simulink model "Non_linear_model_step_response_small_large"  (R2021b)
settings: Solver=FixedStepAuto  StartTime=0.0  StopTime=30  FixedStep=0.001  RelTol=1e-3  EnableMultiTasking=on
undefined symbols (not defined in the file): F_js, F_s, LF, LF_j, LT_i, LT_ji, SF, SF_j, ST_i, ST_ji, T_is, T_jis, T_js, T_s
settings Model: Creator=Administrator  LastModifiedBy=Administrator

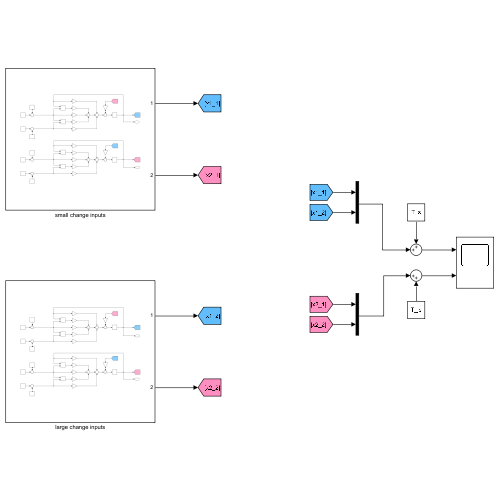
[thumbnail: Simulink's stored preview of the top-level diagram]
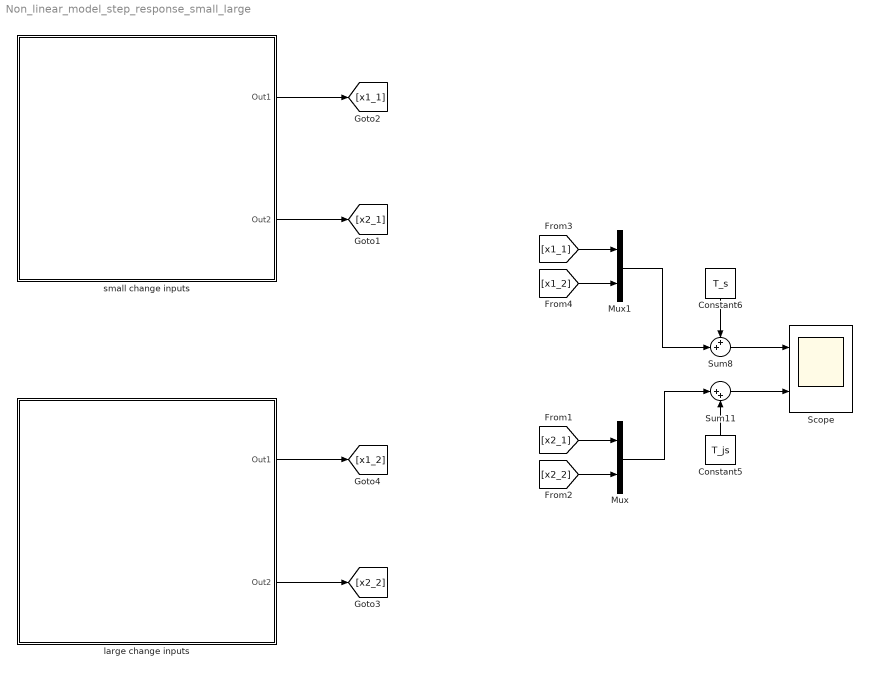
== system Non_linear_model_step_response_small_large ==
  Constant5 : Constant  Value=T_js
  Constant6 : Constant  Value=T_s
  Mux : Mux  Inputs=2
  Mux1 : Mux  Inputs=2
  Scope : Scope  NumInputPorts=2
  Sum11 : Sum  Inputs=|++
  Sum8 : Sum  Inputs=++|
  large change inputs : Subsystem
  small change inputs : Subsystem
  wires:
  Mux1/1 -> Sum8/2
  Sum8/1 -> Scope/1
  Sum11/1 -> Scope/2
  Mux/1 -> Sum11/1
  Constant5/1 -> Sum11/2
  Constant6/1 -> Sum8/1
  small change inputs/1(Out1) -> [x1_1]
  small change inputs/2(Out2) -> [x2_1]
  large change inputs/2(Out2) -> [x2_2]
  large change inputs/1(Out1) -> [x1_2]
  [x2_2] -> Mux/2
  [x2_1] -> Mux/1
  [x1_1] -> Mux1/1
  [x1_2] -> Mux1/2

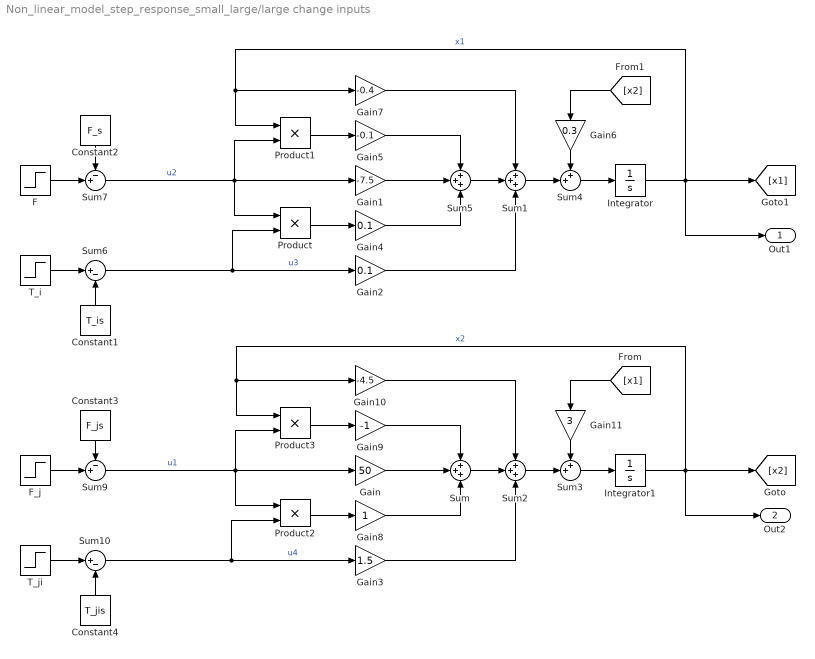
== system Non_linear_model_step_response_small_large/large change inputs ==
  Constant1 : Constant  Value=T_is
  Constant2 : Constant  Value=F_s
  Constant3 : Constant  Value=F_js
  Constant4 : Constant  Value=T_jis
  F : Step  Time=0  After=LF  SampleTime=0
  F_j : Step  Time=0  After=LF_j  SampleTime=0
  Gain : Gain  Gain=50
  Gain1 : Gain  Gain=-7.5
  Gain10 : Gain  Gain=-4.5
  Gain11 : Gain  Gain=3
  Gain2 : Gain  Gain=0.1
  Gain3 : Gain  Gain=1.5
  Gain4 : Gain  Gain=0.1
  Gain5 : Gain  Gain=-0.1
  Gain6 : Gain  Gain=0.3
  Gain7 : Gain  Gain=-0.4
  Gain8 : Gain
  Gain9 : Gain  Gain=-1
  Integrator : Integrator
  Integrator1 : Integrator
  Product{,1..3} (4 alike) : Product
  Sum{,1..2,5} (4 alike) : Sum  Inputs=+++
  Sum10 : Sum  Inputs=|+-
  Sum3 : Sum  Inputs=++|
  Sum4 : Sum  Inputs=++|
  Sum6 : Sum  Inputs=|+-
  Sum7 : Sum  Inputs=-+|
  Sum9 : Sum  Inputs=-+|
  T_i : Step  Time=0  After=LT_i  SampleTime=0
  T_ji : Step  Time=0  After=LT_ji  SampleTime=0
  Out1 : Outport
  Out2 : Outport  Port=2
  wires:
  T_ji/1 -> Sum10/1
  Gain6/1 -> Sum4/1
  Sum6/1 -> Gain2/1, Product/2  "u3"
  Sum7/1 -> Product1/2, Gain1/1, Product/1  "u2"
  T_i/1 -> Sum6/1
  Product3/1 -> Gain9/1
  Constant4/1 -> Sum10/2
  Gain7/1 -> Sum1/1
  F_j/1 -> Sum9/2
  Sum10/1 -> Gain3/1, Product2/2  "u4"
  Sum2/1 -> Sum3/2
  F/1 -> Sum7/2
  Constant2/1 -> Sum7/1
  Sum3/1 -> Integrator1/1
  Sum/1 -> Sum2/2
  Product1/1 -> Gain5/1
  Gain9/1 -> Sum/1
  Product2/1 -> Gain8/1
  Gain8/1 -> Sum/3
  Constant1/1 -> Sum6/2
  [x2] -> Gain6/1
  Sum1/1 -> Sum4/2
  Constant3/1 -> Sum9/1
  Integrator/1 -> Out1/1, [x1], Gain7/1, Product1/1  "x1"
  Gain5/1 -> Sum5/1
  Sum4/1 -> Integrator/1
  Gain11/1 -> Sum3/1
  Gain3/1 -> Sum2/3
  Sum5/1 -> Sum1/2
  Sum9/1 -> Gain/1, Product3/2, Product2/1  "u1"
  Gain1/1 -> Sum5/2
  Gain10/1 -> Sum2/1
  Integrator1/1 -> Out2/1, [x2], Gain10/1, Product3/1  "x2"
  [x1] -> Gain11/1
  Gain4/1 -> Sum5/3
  Gain2/1 -> Sum1/3
  Product/1 -> Gain4/1
  Gain/1 -> Sum/2

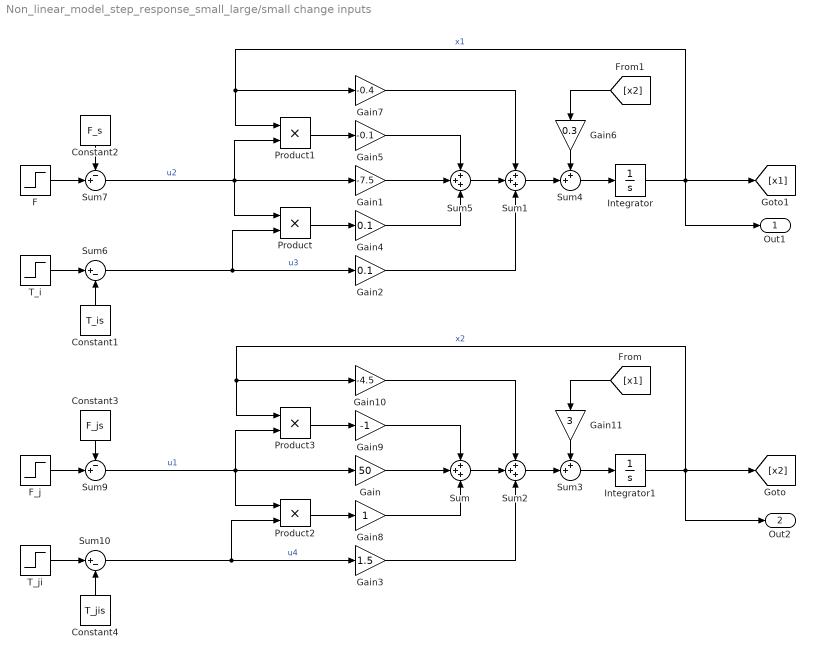
== system Non_linear_model_step_response_small_large/small change inputs ==
  Constant1 : Constant  Value=T_is
  Constant2 : Constant  Value=F_s
  Constant3 : Constant  Value=F_js
  Constant4 : Constant  Value=T_jis
  F : Step  Time=0  After=SF  SampleTime=0
  F_j : Step  Time=0  After=SF_j  SampleTime=0
  Gain : Gain  Gain=50
  Gain1 : Gain  Gain=-7.5
  Gain10 : Gain  Gain=-4.5
  Gain11 : Gain  Gain=3
  Gain2 : Gain  Gain=0.1
  Gain3 : Gain  Gain=1.5
  Gain4 : Gain  Gain=0.1
  Gain5 : Gain  Gain=-0.1
  Gain6 : Gain  Gain=0.3
  Gain7 : Gain  Gain=-0.4
  Gain8 : Gain
  Gain9 : Gain  Gain=-1
  Integrator : Integrator
  Integrator1 : Integrator
  Product{,1..3} (4 alike) : Product
  Sum{,1..2,5} (4 alike) : Sum  Inputs=+++
  Sum10 : Sum  Inputs=|+-
  Sum3 : Sum  Inputs=++|
  Sum4 : Sum  Inputs=++|
  Sum6 : Sum  Inputs=|+-
  Sum7 : Sum  Inputs=-+|
  Sum9 : Sum  Inputs=-+|
  T_i : Step  Time=0  After=ST_i  SampleTime=0
  T_ji : Step  Time=0  After=ST_ji  SampleTime=0
  Out1 : Outport
  Out2 : Outport  Port=2
  wires:
  Gain/1 -> Sum/2
  Product/1 -> Gain4/1
  Gain2/1 -> Sum1/3
  Gain4/1 -> Sum5/3
  [x1] -> Gain11/1
  Integrator1/1 -> Out2/1, Product3/1, Gain10/1, [x2]  "x2"
  Gain10/1 -> Sum2/1
  Gain1/1 -> Sum5/2
  Sum9/1 -> Product2/1, Product3/2, Gain/1  "u1"
  Sum5/1 -> Sum1/2
  Gain3/1 -> Sum2/3
  Gain11/1 -> Sum3/1
  Sum4/1 -> Integrator/1
  Gain5/1 -> Sum5/1
  Integrator/1 -> Out1/1, Product1/1, Gain7/1, [x1]  "x1"
  Constant3/1 -> Sum9/1
  Sum1/1 -> Sum4/2
  [x2] -> Gain6/1
  Constant1/1 -> Sum6/2
  Gain8/1 -> Sum/3
  Product2/1 -> Gain8/1
  Gain9/1 -> Sum/1
  Product1/1 -> Gain5/1
  Sum/1 -> Sum2/2
  Sum3/1 -> Integrator1/1
  Constant2/1 -> Sum7/1
  F/1 -> Sum7/2
  Sum2/1 -> Sum3/2
  Sum10/1 -> Product2/2, Gain3/1  "u4"
  F_j/1 -> Sum9/2
  Gain7/1 -> Sum1/1
  Constant4/1 -> Sum10/2
  Product3/1 -> Gain9/1
  T_i/1 -> Sum6/1
  Sum7/1 -> Product/1, Gain1/1, Product1/2  "u2"
  Sum6/1 -> Product/2, Gain2/1  "u3"
  Gain6/1 -> Sum4/1
  T_ji/1 -> Sum10/1
